simulink model "facilRkk4_simul"  (R2025a)
settings: Solver=VariableStepAuto  StartTime=0.0  StopTime=10.0  RelTol=1e-3
values from neighbouring files (symbols this model uses):
  h = 0.1    [ejemplo_NOlineal_RK4.m]    (also in euler_explicita.m = (tf - t0)/n; euler_explicito.m = (tf - t0)/n; euler_midpoint.m = (tf - t0)/n; examplecrk4.m)
  y0 = 1    [ExampleEuler.m]    (also in ejemplo_NOlineal_RK4.m; examplecrk4.m; exmapleEuler2.m; lineal_RK4.m)
settings Model: Creator=a.diteodoro  LastModifiedBy=a.diteodoro

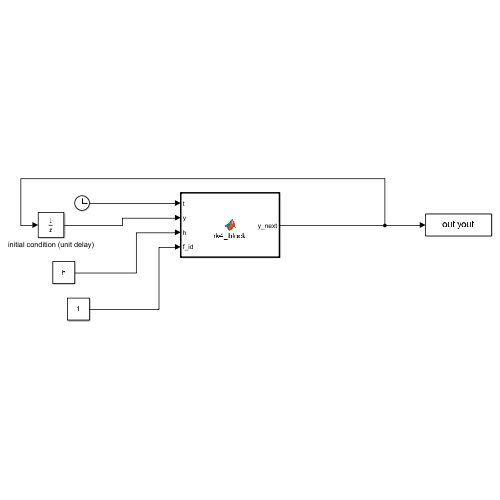
[thumbnail: Simulink's stored preview of the top-level diagram]
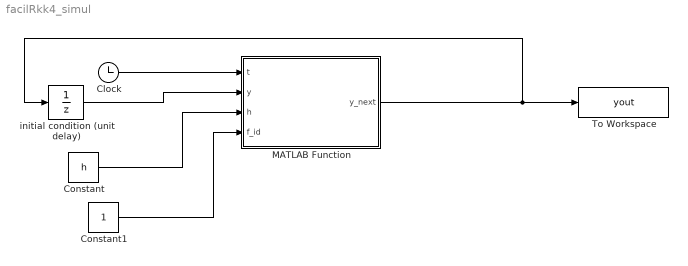
== system facilRkk4_simul ==
  Clock : Clock
  Constant : Constant  Value=h
  Constant1 : Constant
  MATLAB Function : MATLAB Function  TreatAsAtomicUnit=on
  To Workspace : ToWorkspace  VariableName=yout  SaveFormat=Structure With Time  SampleTime=-1
  initial condition (unit delay) : UnitDelay  InitialCondition=y0  SampleTime=-1  HasFrameUpgradeWarning=on
  wires:
  initial condition (unit delay)/1 -> MATLAB Function/2(y)
  Clock/1 -> MATLAB Function/1(t)
  Constant/1 -> MATLAB Function/3(h)
  MATLAB Function/1(y_next) -> initial condition (unit delay)/1, To Workspace/1
  Constant1/1 -> MATLAB Function/4(f_id)

== matlab function facilRkk4_simul/MATLAB Function ==
  data: t input; y_next output; y input; h input; f_id input
function y_next = rk4_block(t, y, h, f_id)
%#codegen

% RK4 con selector de funcion

switch f_id
    case 1
        k1 = y;
        k2 = y + h*k1/2;
        k3 = y + h*k2/2;
        k4 = y + h*k3;

    case 2
        k1 = t^2 + y;
        k2 = (t+h/2)^2 + (y + h*k1/2);
        k3 = (t+h/2)^2 + (y + h*k2/2);
        k4 = (t+h)^2 + (y + h*k3);

    otherwise
        k1 = y;
        k2 = y;
        k3 = y;
        k4 = y;
end

y_next = y + (h/6)*(k1 + 2*k2 + 2*k3 + k4);
